simulink model "Delay"  (R2014b)
settings: Solver=ode45  StartTime=0.0  StopTime=10.0  RelTol=1e-3
libraries: dspsigops x1, dspvision x1, dspsnks4 x1
settings Model: Creator=ICLab  LastModifiedBy=ICLab
settings OptimizationCC: OptimizeModelRefInitCode=on  LifeSpan=1
settings RTWCC: SystemTargetFile=ert.tlc  GenCodeOnly=on  TemplateMakefile=ert_default_tmf  Description=Embedded Coder  ProcessScript=ert_make_rtw_hook
settings CodeAppCC: IgnoreCustomStorageClasses=off
settings ERTTargetCC: CodeReplacementLibrary=ARM Cortex-M  GenerateSampleERTMain=on  ERTCustomFileTemplate=example_file_process.tlc

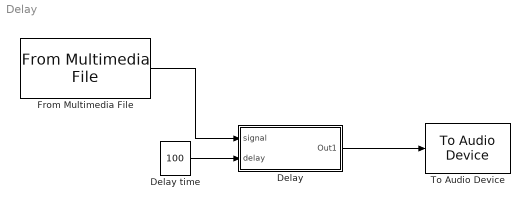
== system Delay ==
  Delay : Subsystem
  Delay time : Constant  Value=100  VectorParams1D=off
  From Multimedia File : dspvision/From Multimedia File  inputFilename=C:\Users\ICLab\Desktop\Embedded system\MATLAB_DSP\distortion\harmonyChorus.wav  loop=on  numPlays=inf  outputStreams=Audio only  videoDataType=single  audioDataType=double  inheritSampleTime=on  userDefinedSampleTime=1/30  noAudioOutput=off  isIntensityVideo=off  fourcc=RGB  colorVideoFormat=Separate color signals  outputEOF=off  dataOrg=Column-major  audioFrameSize=2048  computeAudioFrameSize=off  outSamplingMode=Sample based
  To Audio Device : dspsnks4/To Audio Device  deviceName=Default  inheritSampleRate=on  sampleRate=44100  deviceDatatype=Determine from input data type  autoBufferSize=on  bufferSize=4096  queueDuration=1.0  defaultOutputChannelMapping=on  outputChannelMapping=1:2  outputNumUnderrunSamples=off
  wires:
  From Multimedia File/1 -> Delay/1(signal)
  Delay/1(Out1) -> To Audio Device/1
  Delay time/1 -> Delay/2("delay ")

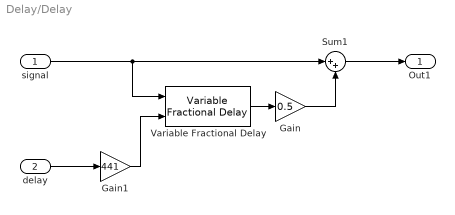
== system Delay/Delay ==
  signal : Inport
  "delay " : Inport  Port=2
  Gain : Gain  Gain=0.5
  Gain1 : Gain  Gain=441
  Sum1 : Sum  Inputs=|++
  Variable Fractional Delay : dspsigops/Variable Fractional Delay  mode=OBSOLETE  modeActive=Linear  dmax=44100  InputProcessing=Columns as channels (frame based)  L=4  FarrowL=4  R=10  alpha=1  ic=0  fallbackFIR=Clip to the minimum value necessary for centered kernel  fallbackFarrow=Clip to the minimum value necessary for centered kernel  noDFT=off  roundingMode=Zero  overflowMode=off
  Out1 : Outport
  wires:
  Sum1/1 -> Out1/1
  signal/1 -> Sum1/1, Variable Fractional Delay/1
  Variable Fractional Delay/1 -> Gain/1
  Gain/1 -> Sum1/2
  "delay "/1 -> Gain1/1
  Gain1/1 -> Variable Fractional Delay/2
